simulink model "Quadcopter_LQR_PI_Observer_6DOF"  (R2022a)
settings: Solver=VariableStepAuto  StartTime=0.0  StopTime=25  RelTol=1e-3
undefined symbols (not defined in the file): A, B, C, Klqr, L
settings Model: Creator=creec  LastModifiedBy=creec

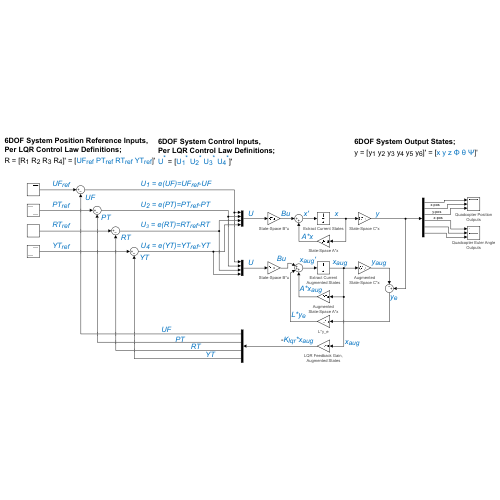
[thumbnail: Simulink's stored preview of the top-level diagram]
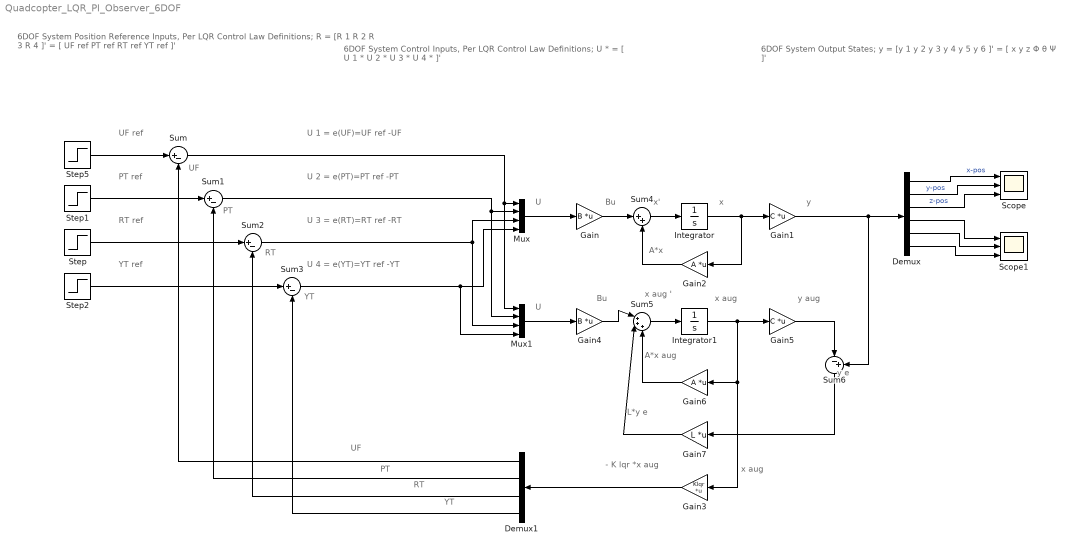
== system Quadcopter_LQR_PI_Observer_6DOF ==
  note: PT
  note: y
  note: U 3 = e(RT)=RT ref -RT
  note: U 4 = e(YT)=YT ref -YT
  note: 6DOF System Control Inputs,
      | Per LQR Control Law Definitions;
      | U * = [ U 1 * U 2 * U 3 * U 4 * ]'
  note: U 2 = e(PT)=PT ref -PT
  note: RT
  note: PT
  note: 6DOF System Position Reference Inputs,
      | Per LQR Control Law Definitions;
      | R = [R 1 R 2 R 3 R 4 ]' = [ UF ref PT ref RT ref YT ref ]'
  note: - K lqr *x aug
  note: UF
  note: Bu
  note: UF ref
  note: U 1 = e(UF)=UF ref -UF
  note: RT ref
  note: x
  note: UF
  note: A*x
  note: YT ref
  note: PT ref
  note: U
  note: x'
  note: YT
  note: RT
  note: YT
  note: x aug
  note: U
  note: x aug '
  note: A*x aug
  note: Bu
  note: 6DOF System Output States;
      | y = [y 1 y 2 y 3 y 4 y 5 y 6 ]' = [ x y z Φ θ Ψ ]'
  note: y aug
  note: y e
  note: L*y e
  note: x aug
  Demux : Demux  Outputs=6
  Demux1 : Demux
  Gain : Gain  Gain=B  Multiplication=Matrix(K*u)
      settings: AttributesFormatString=State-Space B*u
  Gain1 : Gain  Gain=C  Multiplication=Matrix(K*u)
      settings: AttributesFormatString=State-Space C*x
  Gain2 : Gain  Gain=A  Multiplication=Matrix(K*u)
      settings: AttributesFormatString=State-Space A*x
  Gain3 : Gain  Gain=Klqr  Multiplication=Matrix(K*u)
      settings: AttributesFormatString=|
      | LQR Feedback Gain,
      | Augmented States
  Gain4 : Gain  Gain=B  Multiplication=Matrix(K*u)
      settings: AttributesFormatString=State-Space B*u
  Gain5 : Gain  Gain=C  Multiplication=Matrix(K*u)
      settings: AttributesFormatString=|
      | Augmented
      | State-Space C*x
  Gain6 : Gain  Gain=A  Multiplication=Matrix(K*u)
      settings: AttributesFormatString=|
      | Augmented
      | State-Space A*x
  Gain7 : Gain  Gain=L  Multiplication=Matrix(K*u)
      settings: AttributesFormatString=L*y_e
  Integrator : Integrator
      settings: AttributesFormatString=Extract Current States
  Integrator1 : Integrator
      settings: AttributesFormatString=|
      | Extract Current
      | Augmented States
  Mux : Mux
  Mux1 : Mux
  Scope : Scope  NumInputPorts=3
      settings: AttributesFormatString=|
      | Quadcopter Position
      | Outputs
  Scope1 : Scope  NumInputPorts=3
      settings: AttributesFormatString=|
      | Quadcopter Euler Angle
      | Outputs
  Step : Step  Time=15  After=1.5  SampleTime=0
  Step1 : Step  Time=10  After=-2  SampleTime=0
  Step2 : Step  Time=12  After=1.5  SampleTime=0
  Step5 : Step  SampleTime=0
  Sum{,1..3} (4 alike) : Sum  Inputs=|+-
  Sum4 : Sum  Inputs=|++
  Sum5 : Sum  Inputs=|+++
  Sum6 : Sum  Inputs=|-+
  wires:
  Gain1/1 -> Sum6/2, Demux/1
  Sum1/1 -> Mux/2, Mux1/2
  Demux1/3 -> Sum2/2
  Sum2/1 -> Mux/3, Mux1/3
  Demux1/2 -> Sum1/2
  Demux/5 -> Scope1/2
  Step1/1 -> Sum1/1
  Step/1 -> Sum2/1
  Gain3/1 -> Demux1/1
  Demux/6 -> Scope1/3
  Step2/1 -> Sum3/1
  Gain/1 -> Sum4/1
  Demux1/1 -> Sum/2
  Sum3/1 -> Mux/4, Mux1/4
  Demux/1 -> Scope/1  "x-pos"
  Demux/3 -> Scope/3  "z-pos"
  Gain2/1 -> Sum4/2
  Sum4/1 -> Integrator/1
  Demux/4 -> Scope1/1
  Integrator/1 -> Gain2/1, Gain1/1
  Mux/1 -> Gain/1
  Demux/2 -> Scope/2  "y-pos"
  Demux1/4 -> Sum3/2
  Step5/1 -> Sum/1
  Sum/1 -> Mux1/1, Mux/1
  Mux1/1 -> Gain4/1
  Sum5/1 -> Integrator1/1
  Gain4/1 -> Sum5/1
  Gain5/1 -> Sum6/1
  Integrator1/1 -> Gain3/1, Gain6/1, Gain5/1
  Gain6/1 -> Sum5/3
  Gain7/1 -> Sum5/2
  Sum6/1 -> Gain7/1
